simulink model "vocoder_model"  (R2017b)
settings: Solver=VariableStepAuto  StartTime=0.0  StopTime=20  RelTol=1e-3
undefined symbols (not defined in the file or in its folder): NB
libraries: xbsIndex_r4 x1026, dspsrcs4 x1
(part 2 of 8)

== system vocoder_model/Channel_25 ==
  Input : Inport
  Abs Scope : Scope
  Absolute : xbsIndex_r4/Absolute  precision=User Defined  arith_type="Signed  (2's comp)"  n_bits=16  bin_pt=15  quantization=Truncate  overflow=Wrap  en=off  latency=0  dbl_ovrd=off  block_type=abs
  Convert : xbsIndex_r4/Convert  gui_display_data_type=Fixed-point  arith_type="Signed  (2's comp)"  n_bits=16  bin_pt=15  float_type=Single  exp_bits=8  fraction_bits=24  quantization=Truncate  overflow=Wrap  en=off  latency=0  pipeline=off  dbl_ovrd=off  block_type=convert
  Final Channel Scope : Scope
  Gateway In : xbsIndex_r4/Gateway In  gui_display_data_type=Fixed-point  arith_type="Signed  (2's comp)"  n_bits=16  bin_pt=15  preci_type=Single  exp_width=8  frac_width=24  rows=1  columns=1  quantization=Truncate  overflow=Wrap  period=1/8000  UseAsADC=off  ADCChannel='1'  interface=None  automatic_assignment=on  address_offset=hex2dec('00')  intf_name=''  intf_description=''  default_value=0  timing_constraint=None  locs_specified=off  LOCs={}  io_standard={}  inherit_from_input=off  hdl_port=on  dbl_ovrd=off  block_type=gatewayin
  Gateway Out{,1..3} (4 alike) : xbsIndex_r4/Gateway Out  inherit_from_input=off  hdl_port=off  rows=1  columns=1  UseAsDAC=off  DACChannel='1'  interface=None  automatic_assignment=on  address_offset=hex2dec('00')  intf_name=''  intf_description=''  timing_constraint=None  locs_specified=off  LOCs={}  io_standard={}  block_type=gatewayout
  IIR Filter : Subsystem
  IIR Filter Scope : Scope
  LPF Scope : Scope
  Low Pass Filter : Subsystem
  Mult : xbsIndex_r4/Mult  precision=User Defined  arith_type="Signed  (2's comp)"  n_bits=16  bin_pt=15  quantization=Truncate  overflow=Wrap  en=off  latency=0  use_behavioral_HDL=off  opt=Speed  use_embedded=on  optimum_pipeline=off  pipeline=on  dbl_ovrd=off  use_rpm=on  placement_style=Triangular  block_type=mult
  Sine Wave : Sin  Frequency=2*pi*fc  SampleTime=1/8000
  Output : Outport
  wires:
  Input/1 -> IIR Filter/1(Input)
  IIR Filter/1(Output) -> Gateway Out1/1, Absolute/1
  Sine Wave/1 -> Gateway In/1
  Convert/1 -> Mult/1
  Gateway In/1 -> Mult/2
  Absolute/1 -> Gateway Out2/1, Low Pass Filter/1(Input1)
  Low Pass Filter/1(Output1) -> Gateway Out3/1, Convert/1
  Gateway Out/1 -> Output/1, Final Channel Scope/1
  Mult/1 -> Gateway Out/1
  Gateway Out1/1 -> IIR Filter Scope/1
  Gateway Out2/1 -> Abs Scope/1
  Gateway Out3/1 -> LPF Scope/1

== system vocoder_model/Channel_26 ==
  Input : Inport
  Abs Scope : Scope
  Absolute : xbsIndex_r4/Absolute  precision=User Defined  arith_type="Signed  (2's comp)"  n_bits=16  bin_pt=15  quantization=Truncate  overflow=Wrap  en=off  latency=0  dbl_ovrd=off  block_type=abs
  Convert : xbsIndex_r4/Convert  gui_display_data_type=Fixed-point  arith_type="Signed  (2's comp)"  n_bits=16  bin_pt=15  float_type=Single  exp_bits=8  fraction_bits=24  quantization=Truncate  overflow=Wrap  en=off  latency=0  pipeline=off  dbl_ovrd=off  block_type=convert
  Final Channel Scope : Scope
  Gateway In : xbsIndex_r4/Gateway In  gui_display_data_type=Fixed-point  arith_type="Signed  (2's comp)"  n_bits=16  bin_pt=15  preci_type=Single  exp_width=8  frac_width=24  rows=1  columns=1  quantization=Truncate  overflow=Wrap  period=1/8000  UseAsADC=off  ADCChannel='1'  interface=None  automatic_assignment=on  address_offset=hex2dec('00')  intf_name=''  intf_description=''  default_value=0  timing_constraint=None  locs_specified=off  LOCs={}  io_standard={}  inherit_from_input=off  hdl_port=on  dbl_ovrd=off  block_type=gatewayin
  Gateway Out{,1..3} (4 alike) : xbsIndex_r4/Gateway Out  inherit_from_input=off  hdl_port=off  rows=1  columns=1  UseAsDAC=off  DACChannel='1'  interface=None  automatic_assignment=on  address_offset=hex2dec('00')  intf_name=''  intf_description=''  timing_constraint=None  locs_specified=off  LOCs={}  io_standard={}  block_type=gatewayout
  IIR Filter : Subsystem
  IIR Filter Scope : Scope
  LPF Scope : Scope
  Low Pass Filter : Subsystem
  Mult : xbsIndex_r4/Mult  precision=User Defined  arith_type="Signed  (2's comp)"  n_bits=16  bin_pt=15  quantization=Truncate  overflow=Wrap  en=off  latency=0  use_behavioral_HDL=off  opt=Speed  use_embedded=on  optimum_pipeline=off  pipeline=on  dbl_ovrd=off  use_rpm=on  placement_style=Triangular  block_type=mult
  Sine Wave : Sin  Frequency=2*pi*fc  SampleTime=1/8000
  Output : Outport
  wires:
  Input/1 -> IIR Filter/1(Input)
  IIR Filter/1(Output) -> Gateway Out1/1, Absolute/1
  Sine Wave/1 -> Gateway In/1
  Convert/1 -> Mult/1
  Gateway In/1 -> Mult/2
  Absolute/1 -> Gateway Out2/1, Low Pass Filter/1(Input1)
  Low Pass Filter/1(Output1) -> Gateway Out3/1, Convert/1
  Gateway Out/1 -> Output/1, Final Channel Scope/1
  Mult/1 -> Gateway Out/1
  Gateway Out1/1 -> IIR Filter Scope/1
  Gateway Out2/1 -> Abs Scope/1
  Gateway Out3/1 -> LPF Scope/1

== system vocoder_model/Channel_27 ==
  Input : Inport
  Abs Scope : Scope
  Absolute : xbsIndex_r4/Absolute  precision=User Defined  arith_type="Signed  (2's comp)"  n_bits=16  bin_pt=15  quantization=Truncate  overflow=Wrap  en=off  latency=0  dbl_ovrd=off  block_type=abs
  Convert : xbsIndex_r4/Convert  gui_display_data_type=Fixed-point  arith_type="Signed  (2's comp)"  n_bits=16  bin_pt=15  float_type=Single  exp_bits=8  fraction_bits=24  quantization=Truncate  overflow=Wrap  en=off  latency=0  pipeline=off  dbl_ovrd=off  block_type=convert
  Final Channel Scope : Scope
  Gateway In : xbsIndex_r4/Gateway In  gui_display_data_type=Fixed-point  arith_type="Signed  (2's comp)"  n_bits=16  bin_pt=15  preci_type=Single  exp_width=8  frac_width=24  rows=1  columns=1  quantization=Truncate  overflow=Wrap  period=1/8000  UseAsADC=off  ADCChannel='1'  interface=None  automatic_assignment=on  address_offset=hex2dec('00')  intf_name=''  intf_description=''  default_value=0  timing_constraint=None  locs_specified=off  LOCs={}  io_standard={}  inherit_from_input=off  hdl_port=on  dbl_ovrd=off  block_type=gatewayin
  Gateway Out{,1..3} (4 alike) : xbsIndex_r4/Gateway Out  inherit_from_input=off  hdl_port=off  rows=1  columns=1  UseAsDAC=off  DACChannel='1'  interface=None  automatic_assignment=on  address_offset=hex2dec('00')  intf_name=''  intf_description=''  timing_constraint=None  locs_specified=off  LOCs={}  io_standard={}  block_type=gatewayout
  IIR Filter : Subsystem
  IIR Filter Scope : Scope
  LPF Scope : Scope
  Low Pass Filter : Subsystem
  Mult : xbsIndex_r4/Mult  precision=User Defined  arith_type="Signed  (2's comp)"  n_bits=16  bin_pt=15  quantization=Truncate  overflow=Wrap  en=off  latency=0  use_behavioral_HDL=off  opt=Speed  use_embedded=on  optimum_pipeline=off  pipeline=on  dbl_ovrd=off  use_rpm=on  placement_style=Triangular  block_type=mult
  Sine Wave : Sin  Frequency=2*pi*fc  SampleTime=1/8000
  Output : Outport
  wires:
  Input/1 -> IIR Filter/1(Input)
  IIR Filter/1(Output) -> Gateway Out1/1, Absolute/1
  Sine Wave/1 -> Gateway In/1
  Convert/1 -> Mult/1
  Gateway In/1 -> Mult/2
  Absolute/1 -> Gateway Out2/1, Low Pass Filter/1(Input1)
  Low Pass Filter/1(Output1) -> Gateway Out3/1, Convert/1
  Gateway Out/1 -> Output/1, Final Channel Scope/1
  Mult/1 -> Gateway Out/1
  Gateway Out1/1 -> IIR Filter Scope/1
  Gateway Out2/1 -> Abs Scope/1
  Gateway Out3/1 -> LPF Scope/1

== system vocoder_model/Channel_28 ==
  Input : Inport
  Abs Scope : Scope
  Absolute : xbsIndex_r4/Absolute  precision=User Defined  arith_type="Signed  (2's comp)"  n_bits=16  bin_pt=15  quantization=Truncate  overflow=Wrap  en=off  latency=0  dbl_ovrd=off  block_type=abs
  Convert : xbsIndex_r4/Convert  gui_display_data_type=Fixed-point  arith_type="Signed  (2's comp)"  n_bits=16  bin_pt=15  float_type=Single  exp_bits=8  fraction_bits=24  quantization=Truncate  overflow=Wrap  en=off  latency=0  pipeline=off  dbl_ovrd=off  block_type=convert
  Final Channel Scope : Scope
  Gateway In : xbsIndex_r4/Gateway In  gui_display_data_type=Fixed-point  arith_type="Signed  (2's comp)"  n_bits=16  bin_pt=15  preci_type=Single  exp_width=8  frac_width=24  rows=1  columns=1  quantization=Truncate  overflow=Wrap  period=1/8000  UseAsADC=off  ADCChannel='1'  interface=None  automatic_assignment=on  address_offset=hex2dec('00')  intf_name=''  intf_description=''  default_value=0  timing_constraint=None  locs_specified=off  LOCs={}  io_standard={}  inherit_from_input=off  hdl_port=on  dbl_ovrd=off  block_type=gatewayin
  Gateway Out{,1..3} (4 alike) : xbsIndex_r4/Gateway Out  inherit_from_input=off  hdl_port=off  rows=1  columns=1  UseAsDAC=off  DACChannel='1'  interface=None  automatic_assignment=on  address_offset=hex2dec('00')  intf_name=''  intf_description=''  timing_constraint=None  locs_specified=off  LOCs={}  io_standard={}  block_type=gatewayout
  IIR Filter : Subsystem
  IIR Filter Scope : Scope
  LPF Scope : Scope
  Low Pass Filter : Subsystem
  Mult : xbsIndex_r4/Mult  precision=User Defined  arith_type="Signed  (2's comp)"  n_bits=16  bin_pt=15  quantization=Truncate  overflow=Wrap  en=off  latency=0  use_behavioral_HDL=off  opt=Speed  use_embedded=on  optimum_pipeline=off  pipeline=on  dbl_ovrd=off  use_rpm=on  placement_style=Triangular  block_type=mult
  Sine Wave : Sin  Frequency=2*pi*fc  SampleTime=1/8000
  Output : Outport
  wires:
  Input/1 -> IIR Filter/1(Input)
  IIR Filter/1(Output) -> Gateway Out1/1, Absolute/1
  Sine Wave/1 -> Gateway In/1
  Convert/1 -> Mult/1
  Gateway In/1 -> Mult/2
  Absolute/1 -> Gateway Out2/1, Low Pass Filter/1(Input1)
  Low Pass Filter/1(Output1) -> Gateway Out3/1, Convert/1
  Gateway Out/1 -> Output/1, Final Channel Scope/1
  Mult/1 -> Gateway Out/1
  Gateway Out1/1 -> IIR Filter Scope/1
  Gateway Out2/1 -> Abs Scope/1
  Gateway Out3/1 -> LPF Scope/1

== system vocoder_model/Channel_29 ==
  Input : Inport
  Abs Scope : Scope
  Absolute : xbsIndex_r4/Absolute  precision=User Defined  arith_type="Signed  (2's comp)"  n_bits=16  bin_pt=15  quantization=Truncate  overflow=Wrap  en=off  latency=0  dbl_ovrd=off  block_type=abs
  Convert : xbsIndex_r4/Convert  gui_display_data_type=Fixed-point  arith_type="Signed  (2's comp)"  n_bits=16  bin_pt=15  float_type=Single  exp_bits=8  fraction_bits=24  quantization=Truncate  overflow=Wrap  en=off  latency=0  pipeline=off  dbl_ovrd=off  block_type=convert
  Final Channel Scope : Scope
  Gateway In : xbsIndex_r4/Gateway In  gui_display_data_type=Fixed-point  arith_type="Signed  (2's comp)"  n_bits=16  bin_pt=15  preci_type=Single  exp_width=8  frac_width=24  rows=1  columns=1  quantization=Truncate  overflow=Wrap  period=1/8000  UseAsADC=off  ADCChannel='1'  interface=None  automatic_assignment=on  address_offset=hex2dec('00')  intf_name=''  intf_description=''  default_value=0  timing_constraint=None  locs_specified=off  LOCs={}  io_standard={}  inherit_from_input=off  hdl_port=on  dbl_ovrd=off  block_type=gatewayin
  Gateway Out{,1..3} (4 alike) : xbsIndex_r4/Gateway Out  inherit_from_input=off  hdl_port=off  rows=1  columns=1  UseAsDAC=off  DACChannel='1'  interface=None  automatic_assignment=on  address_offset=hex2dec('00')  intf_name=''  intf_description=''  timing_constraint=None  locs_specified=off  LOCs={}  io_standard={}  block_type=gatewayout
  IIR Filter : Subsystem
  IIR Filter Scope : Scope
  LPF Scope : Scope
  Low Pass Filter : Subsystem
  Mult : xbsIndex_r4/Mult  precision=User Defined  arith_type="Signed  (2's comp)"  n_bits=16  bin_pt=15  quantization=Truncate  overflow=Wrap  en=off  latency=0  use_behavioral_HDL=off  opt=Speed  use_embedded=on  optimum_pipeline=off  pipeline=on  dbl_ovrd=off  use_rpm=on  placement_style=Triangular  block_type=mult
  Sine Wave : Sin  Frequency=2*pi*fc  SampleTime=1/8000
  Output : Outport
  wires:
  Input/1 -> IIR Filter/1(Input)
  IIR Filter/1(Output) -> Gateway Out1/1, Absolute/1
  Sine Wave/1 -> Gateway In/1
  Convert/1 -> Mult/1
  Gateway In/1 -> Mult/2
  Absolute/1 -> Gateway Out2/1, Low Pass Filter/1(Input1)
  Low Pass Filter/1(Output1) -> Gateway Out3/1, Convert/1
  Gateway Out/1 -> Output/1, Final Channel Scope/1
  Mult/1 -> Gateway Out/1
  Gateway Out1/1 -> IIR Filter Scope/1
  Gateway Out2/1 -> Abs Scope/1
  Gateway Out3/1 -> LPF Scope/1

== system vocoder_model/Channel_3 ==
  Input : Inport
  Abs Scope : Scope
  Absolute : xbsIndex_r4/Absolute  precision=User Defined  arith_type="Signed  (2's comp)"  n_bits=16  bin_pt=15  quantization=Truncate  overflow=Wrap  en=off  latency=0  dbl_ovrd=off  block_type=abs
  Convert : xbsIndex_r4/Convert  gui_display_data_type=Fixed-point  arith_type="Signed  (2's comp)"  n_bits=16  bin_pt=15  float_type=Single  exp_bits=8  fraction_bits=24  quantization=Truncate  overflow=Wrap  en=off  latency=0  pipeline=off  dbl_ovrd=off  block_type=convert
  Final Channel Scope : Scope
  Gateway In : xbsIndex_r4/Gateway In  gui_display_data_type=Fixed-point  arith_type="Signed  (2's comp)"  n_bits=16  bin_pt=15  preci_type=Single  exp_width=8  frac_width=24  rows=1  columns=1  quantization=Truncate  overflow=Wrap  period=1/8000  UseAsADC=off  ADCChannel='1'  interface=None  automatic_assignment=on  address_offset=hex2dec('00')  intf_name=''  intf_description=''  default_value=0  timing_constraint=None  locs_specified=off  LOCs={}  io_standard={}  inherit_from_input=off  hdl_port=on  dbl_ovrd=off  block_type=gatewayin
  Gateway Out{,1..3} (4 alike) : xbsIndex_r4/Gateway Out  inherit_from_input=off  hdl_port=off  rows=1  columns=1  UseAsDAC=off  DACChannel='1'  interface=None  automatic_assignment=on  address_offset=hex2dec('00')  intf_name=''  intf_description=''  timing_constraint=None  locs_specified=off  LOCs={}  io_standard={}  block_type=gatewayout
  IIR Filter : Subsystem
  IIR Filter Scope : Scope
  LPF Scope : Scope
  Low Pass Filter : Subsystem
  Mult : xbsIndex_r4/Mult  precision=User Defined  arith_type="Signed  (2's comp)"  n_bits=16  bin_pt=15  quantization=Truncate  overflow=Wrap  en=off  latency=0  use_behavioral_HDL=off  opt=Speed  use_embedded=on  optimum_pipeline=off  pipeline=on  dbl_ovrd=off  use_rpm=on  placement_style=Triangular  block_type=mult
  Sine Wave : Sin  Frequency=2*pi*fc  SampleTime=1/8000
  Output : Outport
  wires:
  Input/1 -> IIR Filter/1(Input)
  IIR Filter/1(Output) -> Gateway Out1/1, Absolute/1
  Sine Wave/1 -> Gateway In/1
  Convert/1 -> Mult/1
  Gateway In/1 -> Mult/2
  Absolute/1 -> Gateway Out2/1, Low Pass Filter/1(Input1)
  Low Pass Filter/1(Output1) -> Gateway Out3/1, Convert/1
  Gateway Out/1 -> Output/1, Final Channel Scope/1
  Mult/1 -> Gateway Out/1
  Gateway Out1/1 -> IIR Filter Scope/1
  Gateway Out2/1 -> Abs Scope/1
  Gateway Out3/1 -> LPF Scope/1

== system vocoder_model/Channel_30 ==
  Input : Inport
  Abs Scope : Scope
  Absolute : xbsIndex_r4/Absolute  precision=User Defined  arith_type="Signed  (2's comp)"  n_bits=16  bin_pt=15  quantization=Truncate  overflow=Wrap  en=off  latency=0  dbl_ovrd=off  block_type=abs
  Convert : xbsIndex_r4/Convert  gui_display_data_type=Fixed-point  arith_type="Signed  (2's comp)"  n_bits=16  bin_pt=15  float_type=Single  exp_bits=8  fraction_bits=24  quantization=Truncate  overflow=Wrap  en=off  latency=0  pipeline=off  dbl_ovrd=off  block_type=convert
  Final Channel Scope : Scope
  Gateway In : xbsIndex_r4/Gateway In  gui_display_data_type=Fixed-point  arith_type="Signed  (2's comp)"  n_bits=16  bin_pt=15  preci_type=Single  exp_width=8  frac_width=24  rows=1  columns=1  quantization=Truncate  overflow=Wrap  period=1/8000  UseAsADC=off  ADCChannel='1'  interface=None  automatic_assignment=on  address_offset=hex2dec('00')  intf_name=''  intf_description=''  default_value=0  timing_constraint=None  locs_specified=off  LOCs={}  io_standard={}  inherit_from_input=off  hdl_port=on  dbl_ovrd=off  block_type=gatewayin
  Gateway Out{,1..3} (4 alike) : xbsIndex_r4/Gateway Out  inherit_from_input=off  hdl_port=off  rows=1  columns=1  UseAsDAC=off  DACChannel='1'  interface=None  automatic_assignment=on  address_offset=hex2dec('00')  intf_name=''  intf_description=''  timing_constraint=None  locs_specified=off  LOCs={}  io_standard={}  block_type=gatewayout
  IIR Filter : Subsystem
  IIR Filter Scope : Scope
  LPF Scope : Scope
  Low Pass Filter : Subsystem
  Mult : xbsIndex_r4/Mult  precision=User Defined  arith_type="Signed  (2's comp)"  n_bits=16  bin_pt=15  quantization=Truncate  overflow=Wrap  en=off  latency=0  use_behavioral_HDL=off  opt=Speed  use_embedded=on  optimum_pipeline=off  pipeline=on  dbl_ovrd=off  use_rpm=on  placement_style=Triangular  block_type=mult
  Sine Wave : Sin  Frequency=2*pi*fc  SampleTime=1/8000
  Output : Outport
  wires:
  Input/1 -> IIR Filter/1(Input)
  IIR Filter/1(Output) -> Gateway Out1/1, Absolute/1
  Sine Wave/1 -> Gateway In/1
  Convert/1 -> Mult/1
  Gateway In/1 -> Mult/2
  Absolute/1 -> Gateway Out2/1, Low Pass Filter/1(Input1)
  Low Pass Filter/1(Output1) -> Gateway Out3/1, Convert/1
  Gateway Out/1 -> Output/1, Final Channel Scope/1
  Mult/1 -> Gateway Out/1
  Gateway Out1/1 -> IIR Filter Scope/1
  Gateway Out2/1 -> Abs Scope/1
  Gateway Out3/1 -> LPF Scope/1

== system vocoder_model/Channel_31 ==
  Input : Inport
  Abs Scope : Scope
  Absolute : xbsIndex_r4/Absolute  precision=User Defined  arith_type="Signed  (2's comp)"  n_bits=16  bin_pt=15  quantization=Truncate  overflow=Wrap  en=off  latency=0  dbl_ovrd=off  block_type=abs
  Convert : xbsIndex_r4/Convert  gui_display_data_type=Fixed-point  arith_type="Signed  (2's comp)"  n_bits=16  bin_pt=15  float_type=Single  exp_bits=8  fraction_bits=24  quantization=Truncate  overflow=Wrap  en=off  latency=0  pipeline=off  dbl_ovrd=off  block_type=convert
  Final Channel Scope : Scope
  Gateway In : xbsIndex_r4/Gateway In  gui_display_data_type=Fixed-point  arith_type="Signed  (2's comp)"  n_bits=16  bin_pt=15  preci_type=Single  exp_width=8  frac_width=24  rows=1  columns=1  quantization=Truncate  overflow=Wrap  period=1/8000  UseAsADC=off  ADCChannel='1'  interface=None  automatic_assignment=on  address_offset=hex2dec('00')  intf_name=''  intf_description=''  default_value=0  timing_constraint=None  locs_specified=off  LOCs={}  io_standard={}  inherit_from_input=off  hdl_port=on  dbl_ovrd=off  block_type=gatewayin
  Gateway Out{,1..3} (4 alike) : xbsIndex_r4/Gateway Out  inherit_from_input=off  hdl_port=off  rows=1  columns=1  UseAsDAC=off  DACChannel='1'  interface=None  automatic_assignment=on  address_offset=hex2dec('00')  intf_name=''  intf_description=''  timing_constraint=None  locs_specified=off  LOCs={}  io_standard={}  block_type=gatewayout
  IIR Filter : Subsystem
  IIR Filter Scope : Scope
  LPF Scope : Scope
  Low Pass Filter : Subsystem
  Mult : xbsIndex_r4/Mult  precision=User Defined  arith_type="Signed  (2's comp)"  n_bits=16  bin_pt=15  quantization=Truncate  overflow=Wrap  en=off  latency=0  use_behavioral_HDL=off  opt=Speed  use_embedded=on  optimum_pipeline=off  pipeline=on  dbl_ovrd=off  use_rpm=on  placement_style=Triangular  block_type=mult
  Sine Wave : Sin  Frequency=2*pi*fc  SampleTime=1/8000
  Output : Outport
  wires:
  Input/1 -> IIR Filter/1(Input)
  IIR Filter/1(Output) -> Gateway Out1/1, Absolute/1
  Sine Wave/1 -> Gateway In/1
  Convert/1 -> Mult/1
  Gateway In/1 -> Mult/2
  Absolute/1 -> Gateway Out2/1, Low Pass Filter/1(Input1)
  Low Pass Filter/1(Output1) -> Gateway Out3/1, Convert/1
  Gateway Out/1 -> Output/1, Final Channel Scope/1
  Mult/1 -> Gateway Out/1
  Gateway Out1/1 -> IIR Filter Scope/1
  Gateway Out2/1 -> Abs Scope/1
  Gateway Out3/1 -> LPF Scope/1

== system vocoder_model/Channel_32 ==
  Input : Inport
  Abs Scope : Scope
  Absolute : xbsIndex_r4/Absolute  precision=User Defined  arith_type="Signed  (2's comp)"  n_bits=16  bin_pt=15  quantization=Truncate  overflow=Wrap  en=off  latency=0  dbl_ovrd=off  block_type=abs
  Convert : xbsIndex_r4/Convert  gui_display_data_type=Fixed-point  arith_type="Signed  (2's comp)"  n_bits=16  bin_pt=15  float_type=Single  exp_bits=8  fraction_bits=24  quantization=Truncate  overflow=Wrap  en=off  latency=0  pipeline=off  dbl_ovrd=off  block_type=convert
  Final Channel Scope : Scope
  Gateway In : xbsIndex_r4/Gateway In  gui_display_data_type=Fixed-point  arith_type="Signed  (2's comp)"  n_bits=16  bin_pt=15  preci_type=Single  exp_width=8  frac_width=24  rows=1  columns=1  quantization=Truncate  overflow=Wrap  period=1/8000  UseAsADC=off  ADCChannel='1'  interface=None  automatic_assignment=on  address_offset=hex2dec('00')  intf_name=''  intf_description=''  default_value=0  timing_constraint=None  locs_specified=off  LOCs={}  io_standard={}  inherit_from_input=off  hdl_port=on  dbl_ovrd=off  block_type=gatewayin
  Gateway Out{,1..3} (4 alike) : xbsIndex_r4/Gateway Out  inherit_from_input=off  hdl_port=off  rows=1  columns=1  UseAsDAC=off  DACChannel='1'  interface=None  automatic_assignment=on  address_offset=hex2dec('00')  intf_name=''  intf_description=''  timing_constraint=None  locs_specified=off  LOCs={}  io_standard={}  block_type=gatewayout
  IIR Filter : Subsystem
  IIR Filter Scope : Scope
  LPF Scope : Scope
  Low Pass Filter : Subsystem
  Mult : xbsIndex_r4/Mult  precision=User Defined  arith_type="Signed  (2's comp)"  n_bits=16  bin_pt=15  quantization=Truncate  overflow=Wrap  en=off  latency=0  use_behavioral_HDL=off  opt=Speed  use_embedded=on  optimum_pipeline=off  pipeline=on  dbl_ovrd=off  use_rpm=on  placement_style=Triangular  block_type=mult
  Sine Wave : Sin  Frequency=2*pi*fc  SampleTime=1/8000
  Output : Outport
  wires:
  Input/1 -> IIR Filter/1(Input)
  IIR Filter/1(Output) -> Gateway Out1/1, Absolute/1
  Sine Wave/1 -> Gateway In/1
  Convert/1 -> Mult/1
  Gateway In/1 -> Mult/2
  Absolute/1 -> Gateway Out2/1, Low Pass Filter/1(Input1)
  Low Pass Filter/1(Output1) -> Gateway Out3/1, Convert/1
  Gateway Out/1 -> Output/1, Final Channel Scope/1
  Mult/1 -> Gateway Out/1
  Gateway Out1/1 -> IIR Filter Scope/1
  Gateway Out2/1 -> Abs Scope/1
  Gateway Out3/1 -> LPF Scope/1

== system vocoder_model/Channel_4 ==
  Input : Inport
  Abs Scope : Scope
  Absolute : xbsIndex_r4/Absolute  precision=User Defined  arith_type="Signed  (2's comp)"  n_bits=16  bin_pt=15  quantization=Truncate  overflow=Wrap  en=off  latency=0  dbl_ovrd=off  block_type=abs
  Convert : xbsIndex_r4/Convert  gui_display_data_type=Fixed-point  arith_type="Signed  (2's comp)"  n_bits=16  bin_pt=15  float_type=Single  exp_bits=8  fraction_bits=24  quantization=Truncate  overflow=Wrap  en=off  latency=0  pipeline=off  dbl_ovrd=off  block_type=convert
  Final Channel Scope : Scope
  Gateway In : xbsIndex_r4/Gateway In  gui_display_data_type=Fixed-point  arith_type="Signed  (2's comp)"  n_bits=16  bin_pt=15  preci_type=Single  exp_width=8  frac_width=24  rows=1  columns=1  quantization=Truncate  overflow=Wrap  period=1/8000  UseAsADC=off  ADCChannel='1'  interface=None  automatic_assignment=on  address_offset=hex2dec('00')  intf_name=''  intf_description=''  default_value=0  timing_constraint=None  locs_specified=off  LOCs={}  io_standard={}  inherit_from_input=off  hdl_port=on  dbl_ovrd=off  block_type=gatewayin
  Gateway Out{,1..3} (4 alike) : xbsIndex_r4/Gateway Out  inherit_from_input=off  hdl_port=off  rows=1  columns=1  UseAsDAC=off  DACChannel='1'  interface=None  automatic_assignment=on  address_offset=hex2dec('00')  intf_name=''  intf_description=''  timing_constraint=None  locs_specified=off  LOCs={}  io_standard={}  block_type=gatewayout
  IIR Filter : Subsystem
  IIR Filter Scope : Scope
  LPF Scope : Scope
  Low Pass Filter : Subsystem
  Mult : xbsIndex_r4/Mult  precision=User Defined  arith_type="Signed  (2's comp)"  n_bits=16  bin_pt=15  quantization=Truncate  overflow=Wrap  en=off  latency=0  use_behavioral_HDL=off  opt=Speed  use_embedded=on  optimum_pipeline=off  pipeline=on  dbl_ovrd=off  use_rpm=on  placement_style=Triangular  block_type=mult
  Sine Wave : Sin  Frequency=2*pi*fc  SampleTime=1/8000
  Output : Outport
  wires:
  Input/1 -> IIR Filter/1(Input)
  IIR Filter/1(Output) -> Gateway Out1/1, Absolute/1
  Sine Wave/1 -> Gateway In/1
  Convert/1 -> Mult/1
  Gateway In/1 -> Mult/2
  Absolute/1 -> Gateway Out2/1, Low Pass Filter/1(Input1)
  Low Pass Filter/1(Output1) -> Gateway Out3/1, Convert/1
  Gateway Out/1 -> Output/1, Final Channel Scope/1
  Mult/1 -> Gateway Out/1
  Gateway Out1/1 -> IIR Filter Scope/1
  Gateway Out2/1 -> Abs Scope/1
  Gateway Out3/1 -> LPF Scope/1

== system vocoder_model/Channel_5 ==
  Input : Inport
  Abs Scope : Scope
  Absolute : xbsIndex_r4/Absolute  precision=User Defined  arith_type="Signed  (2's comp)"  n_bits=16  bin_pt=15  quantization=Truncate  overflow=Wrap  en=off  latency=0  dbl_ovrd=off  block_type=abs
  Convert : xbsIndex_r4/Convert  gui_display_data_type=Fixed-point  arith_type="Signed  (2's comp)"  n_bits=16  bin_pt=15  float_type=Single  exp_bits=8  fraction_bits=24  quantization=Truncate  overflow=Wrap  en=off  latency=0  pipeline=off  dbl_ovrd=off  block_type=convert
  Final Channel Scope : Scope
  Gateway In : xbsIndex_r4/Gateway In  gui_display_data_type=Fixed-point  arith_type="Signed  (2's comp)"  n_bits=16  bin_pt=15  preci_type=Single  exp_width=8  frac_width=24  rows=1  columns=1  quantization=Truncate  overflow=Wrap  period=1/8000  UseAsADC=off  ADCChannel='1'  interface=None  automatic_assignment=on  address_offset=hex2dec('00')  intf_name=''  intf_description=''  default_value=0  timing_constraint=None  locs_specified=off  LOCs={}  io_standard={}  inherit_from_input=off  hdl_port=on  dbl_ovrd=off  block_type=gatewayin
  Gateway Out{,1..3} (4 alike) : xbsIndex_r4/Gateway Out  inherit_from_input=off  hdl_port=off  rows=1  columns=1  UseAsDAC=off  DACChannel='1'  interface=None  automatic_assignment=on  address_offset=hex2dec('00')  intf_name=''  intf_description=''  timing_constraint=None  locs_specified=off  LOCs={}  io_standard={}  block_type=gatewayout
  IIR Filter : Subsystem
  IIR Filter Scope : Scope
  LPF Scope : Scope
  Low Pass Filter : Subsystem
  Mult : xbsIndex_r4/Mult  precision=User Defined  arith_type="Signed  (2's comp)"  n_bits=16  bin_pt=15  quantization=Truncate  overflow=Wrap  en=off  latency=0  use_behavioral_HDL=off  opt=Speed  use_embedded=on  optimum_pipeline=off  pipeline=on  dbl_ovrd=off  use_rpm=on  placement_style=Triangular  block_type=mult
  Sine Wave : Sin  Frequency=2*pi*fc  SampleTime=1/8000
  Output : Outport
  wires:
  Input/1 -> IIR Filter/1(Input)
  IIR Filter/1(Output) -> Gateway Out1/1, Absolute/1
  Sine Wave/1 -> Gateway In/1
  Convert/1 -> Mult/1
  Gateway In/1 -> Mult/2
  Absolute/1 -> Gateway Out2/1, Low Pass Filter/1(Input1)
  Low Pass Filter/1(Output1) -> Gateway Out3/1, Convert/1
  Gateway Out/1 -> Output/1, Final Channel Scope/1
  Mult/1 -> Gateway Out/1
  Gateway Out1/1 -> IIR Filter Scope/1
  Gateway Out2/1 -> Abs Scope/1
  Gateway Out3/1 -> LPF Scope/1

== system vocoder_model/Channel_6 ==
  Input : Inport
  Abs Scope : Scope
  Absolute : xbsIndex_r4/Absolute  precision=User Defined  arith_type="Signed  (2's comp)"  n_bits=16  bin_pt=15  quantization=Truncate  overflow=Wrap  en=off  latency=0  dbl_ovrd=off  block_type=abs
  Convert : xbsIndex_r4/Convert  gui_display_data_type=Fixed-point  arith_type="Signed  (2's comp)"  n_bits=16  bin_pt=15  float_type=Single  exp_bits=8  fraction_bits=24  quantization=Truncate  overflow=Wrap  en=off  latency=0  pipeline=off  dbl_ovrd=off  block_type=convert
  Final Channel Scope : Scope
  Gateway In : xbsIndex_r4/Gateway In  gui_display_data_type=Fixed-point  arith_type="Signed  (2's comp)"  n_bits=16  bin_pt=15  preci_type=Single  exp_width=8  frac_width=24  rows=1  columns=1  quantization=Truncate  overflow=Wrap  period=1/8000  UseAsADC=off  ADCChannel='1'  interface=None  automatic_assignment=on  address_offset=hex2dec('00')  intf_name=''  intf_description=''  default_value=0  timing_constraint=None  locs_specified=off  LOCs={}  io_standard={}  inherit_from_input=off  hdl_port=on  dbl_ovrd=off  block_type=gatewayin
  Gateway Out{,1..3} (4 alike) : xbsIndex_r4/Gateway Out  inherit_from_input=off  hdl_port=off  rows=1  columns=1  UseAsDAC=off  DACChannel='1'  interface=None  automatic_assignment=on  address_offset=hex2dec('00')  intf_name=''  intf_description=''  timing_constraint=None  locs_specified=off  LOCs={}  io_standard={}  block_type=gatewayout
  IIR Filter : Subsystem
  IIR Filter Scope : Scope
  LPF Scope : Scope
  Low Pass Filter : Subsystem
  Mult : xbsIndex_r4/Mult  precision=User Defined  arith_type="Signed  (2's comp)"  n_bits=16  bin_pt=15  quantization=Truncate  overflow=Wrap  en=off  latency=0  use_behavioral_HDL=off  opt=Speed  use_embedded=on  optimum_pipeline=off  pipeline=on  dbl_ovrd=off  use_rpm=on  placement_style=Triangular  block_type=mult
  Sine Wave : Sin  Frequency=2*pi*fc  SampleTime=1/8000
  Output : Outport
  wires:
  Input/1 -> IIR Filter/1(Input)
  IIR Filter/1(Output) -> Gateway Out1/1, Absolute/1
  Sine Wave/1 -> Gateway In/1
  Convert/1 -> Mult/1
  Gateway In/1 -> Mult/2
  Absolute/1 -> Gateway Out2/1, Low Pass Filter/1(Input1)
  Low Pass Filter/1(Output1) -> Gateway Out3/1, Convert/1
  Gateway Out/1 -> Output/1, Final Channel Scope/1
  Mult/1 -> Gateway Out/1
  Gateway Out1/1 -> IIR Filter Scope/1
  Gateway Out2/1 -> Abs Scope/1
  Gateway Out3/1 -> LPF Scope/1

== system vocoder_model/Channel_7 ==
  Input : Inport
  Abs Scope : Scope
  Absolute : xbsIndex_r4/Absolute  precision=User Defined  arith_type="Signed  (2's comp)"  n_bits=16  bin_pt=15  quantization=Truncate  overflow=Wrap  en=off  latency=0  dbl_ovrd=off  block_type=abs
  Convert : xbsIndex_r4/Convert  gui_display_data_type=Fixed-point  arith_type="Signed  (2's comp)"  n_bits=16  bin_pt=15  float_type=Single  exp_bits=8  fraction_bits=24  quantization=Truncate  overflow=Wrap  en=off  latency=0  pipeline=off  dbl_ovrd=off  block_type=convert
  Final Channel Scope : Scope
  Gateway In : xbsIndex_r4/Gateway In  gui_display_data_type=Fixed-point  arith_type="Signed  (2's comp)"  n_bits=16  bin_pt=15  preci_type=Single  exp_width=8  frac_width=24  rows=1  columns=1  quantization=Truncate  overflow=Wrap  period=1/8000  UseAsADC=off  ADCChannel='1'  interface=None  automatic_assignment=on  address_offset=hex2dec('00')  intf_name=''  intf_description=''  default_value=0  timing_constraint=None  locs_specified=off  LOCs={}  io_standard={}  inherit_from_input=off  hdl_port=on  dbl_ovrd=off  block_type=gatewayin
  Gateway Out{,1..3} (4 alike) : xbsIndex_r4/Gateway Out  inherit_from_input=off  hdl_port=off  rows=1  columns=1  UseAsDAC=off  DACChannel='1'  interface=None  automatic_assignment=on  address_offset=hex2dec('00')  intf_name=''  intf_description=''  timing_constraint=None  locs_specified=off  LOCs={}  io_standard={}  block_type=gatewayout
  IIR Filter : Subsystem
  IIR Filter Scope : Scope
  LPF Scope : Scope
  Low Pass Filter : Subsystem
  Mult : xbsIndex_r4/Mult  precision=User Defined  arith_type="Signed  (2's comp)"  n_bits=16  bin_pt=15  quantization=Truncate  overflow=Wrap  en=off  latency=0  use_behavioral_HDL=off  opt=Speed  use_embedded=on  optimum_pipeline=off  pipeline=on  dbl_ovrd=off  use_rpm=on  placement_style=Triangular  block_type=mult
  Sine Wave : Sin  Frequency=2*pi*fc  SampleTime=1/8000
  Output : Outport
  wires:
  Input/1 -> IIR Filter/1(Input)
  IIR Filter/1(Output) -> Gateway Out1/1, Absolute/1
  Sine Wave/1 -> Gateway In/1
  Convert/1 -> Mult/1
  Gateway In/1 -> Mult/2
  Absolute/1 -> Gateway Out2/1, Low Pass Filter/1(Input1)
  Low Pass Filter/1(Output1) -> Gateway Out3/1, Convert/1
  Gateway Out/1 -> Output/1, Final Channel Scope/1
  Mult/1 -> Gateway Out/1
  Gateway Out1/1 -> IIR Filter Scope/1
  Gateway Out2/1 -> Abs Scope/1
  Gateway Out3/1 -> LPF Scope/1

== system vocoder_model/Channel_8 ==
  Input : Inport
  Abs Scope : Scope
  Absolute : xbsIndex_r4/Absolute  precision=User Defined  arith_type="Signed  (2's comp)"  n_bits=16  bin_pt=15  quantization=Truncate  overflow=Wrap  en=off  latency=0  dbl_ovrd=off  block_type=abs
  Convert : xbsIndex_r4/Convert  gui_display_data_type=Fixed-point  arith_type="Signed  (2's comp)"  n_bits=16  bin_pt=15  float_type=Single  exp_bits=8  fraction_bits=24  quantization=Truncate  overflow=Wrap  en=off  latency=0  pipeline=off  dbl_ovrd=off  block_type=convert
  Final Channel Scope : Scope
  Gateway In : xbsIndex_r4/Gateway In  gui_display_data_type=Fixed-point  arith_type="Signed  (2's comp)"  n_bits=16  bin_pt=15  preci_type=Single  exp_width=8  frac_width=24  rows=1  columns=1  quantization=Truncate  overflow=Wrap  period=1/8000  UseAsADC=off  ADCChannel='1'  interface=None  automatic_assignment=on  address_offset=hex2dec('00')  intf_name=''  intf_description=''  default_value=0  timing_constraint=None  locs_specified=off  LOCs={}  io_standard={}  inherit_from_input=off  hdl_port=on  dbl_ovrd=off  block_type=gatewayin
  Gateway Out{,1..3} (4 alike) : xbsIndex_r4/Gateway Out  inherit_from_input=off  hdl_port=off  rows=1  columns=1  UseAsDAC=off  DACChannel='1'  interface=None  automatic_assignment=on  address_offset=hex2dec('00')  intf_name=''  intf_description=''  timing_constraint=None  locs_specified=off  LOCs={}  io_standard={}  block_type=gatewayout
  IIR Filter : Subsystem
  IIR Filter Scope : Scope
  LPF Scope : Scope
  Low Pass Filter : Subsystem
  Mult : xbsIndex_r4/Mult  precision=User Defined  arith_type="Signed  (2's comp)"  n_bits=16  bin_pt=15  quantization=Truncate  overflow=Wrap  en=off  latency=0  use_behavioral_HDL=off  opt=Speed  use_embedded=on  optimum_pipeline=off  pipeline=on  dbl_ovrd=off  use_rpm=on  placement_style=Triangular  block_type=mult
  Sine Wave : Sin  Frequency=2*pi*fc  SampleTime=1/8000
  Output : Outport
  wires:
  Input/1 -> IIR Filter/1(Input)
  IIR Filter/1(Output) -> Gateway Out1/1, Absolute/1
  Sine Wave/1 -> Gateway In/1
  Convert/1 -> Mult/1
  Gateway In/1 -> Mult/2
  Absolute/1 -> Gateway Out2/1, Low Pass Filter/1(Input1)
  Low Pass Filter/1(Output1) -> Gateway Out3/1, Convert/1
  Gateway Out/1 -> Output/1, Final Channel Scope/1
  Mult/1 -> Gateway Out/1
  Gateway Out1/1 -> IIR Filter Scope/1
  Gateway Out2/1 -> Abs Scope/1
  Gateway Out3/1 -> LPF Scope/1

== system vocoder_model/Channel_9 ==
  Input : Inport
  Abs Scope : Scope
  Absolute : xbsIndex_r4/Absolute  precision=User Defined  arith_type="Signed  (2's comp)"  n_bits=16  bin_pt=15  quantization=Truncate  overflow=Wrap  en=off  latency=0  dbl_ovrd=off  block_type=abs
  Convert : xbsIndex_r4/Convert  gui_display_data_type=Fixed-point  arith_type="Signed  (2's comp)"  n_bits=16  bin_pt=15  float_type=Single  exp_bits=8  fraction_bits=24  quantization=Truncate  overflow=Wrap  en=off  latency=0  pipeline=off  dbl_ovrd=off  block_type=convert
  Final Channel Scope : Scope
  Gateway In : xbsIndex_r4/Gateway In  gui_display_data_type=Fixed-point  arith_type="Signed  (2's comp)"  n_bits=16  bin_pt=15  preci_type=Single  exp_width=8  frac_width=24  rows=1  columns=1  quantization=Truncate  overflow=Wrap  period=1/8000  UseAsADC=off  ADCChannel='1'  interface=None  automatic_assignment=on  address_offset=hex2dec('00')  intf_name=''  intf_description=''  default_value=0  timing_constraint=None  locs_specified=off  LOCs={}  io_standard={}  inherit_from_input=off  hdl_port=on  dbl_ovrd=off  block_type=gatewayin
  Gateway Out{,1..3} (4 alike) : xbsIndex_r4/Gateway Out  inherit_from_input=off  hdl_port=off  rows=1  columns=1  UseAsDAC=off  DACChannel='1'  interface=None  automatic_assignment=on  address_offset=hex2dec('00')  intf_name=''  intf_description=''  timing_constraint=None  locs_specified=off  LOCs={}  io_standard={}  block_type=gatewayout
  IIR Filter : Subsystem
  IIR Filter Scope : Scope
  LPF Scope : Scope
  Low Pass Filter : Subsystem
  Mult : xbsIndex_r4/Mult  precision=User Defined  arith_type="Signed  (2's comp)"  n_bits=16  bin_pt=15  quantization=Truncate  overflow=Wrap  en=off  latency=0  use_behavioral_HDL=off  opt=Speed  use_embedded=on  optimum_pipeline=off  pipeline=on  dbl_ovrd=off  use_rpm=on  placement_style=Triangular  block_type=mult
  Sine Wave : Sin  Frequency=2*pi*fc  SampleTime=1/8000
  Output : Outport
  wires:
  Input/1 -> IIR Filter/1(Input)
  IIR Filter/1(Output) -> Gateway Out1/1, Absolute/1
  Sine Wave/1 -> Gateway In/1
  Convert/1 -> Mult/1
  Gateway In/1 -> Mult/2
  Absolute/1 -> Gateway Out2/1, Low Pass Filter/1(Input1)
  Low Pass Filter/1(Output1) -> Gateway Out3/1, Convert/1
  Gateway Out/1 -> Output/1, Final Channel Scope/1
  Mult/1 -> Gateway Out/1
  Gateway Out1/1 -> IIR Filter Scope/1
  Gateway Out2/1 -> Abs Scope/1
  Gateway Out3/1 -> LPF Scope/1

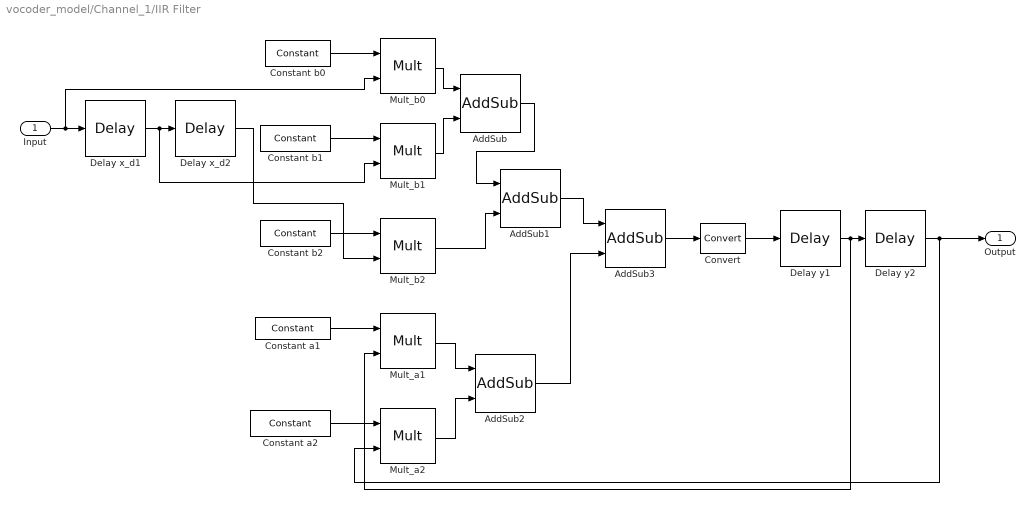
== system vocoder_model/Channel_1/IIR Filter ==
  Input : Inport
  AddSub : xbsIndex_r4/AddSub  mode=Addition  use_carryin=off  use_carryout=off  en=off  latency=0  precision=Full  arith_type=Unsigned  n_bits=16  bin_pt=14  quantization=Truncate  overflow=Wrap  use_behavioral_HDL=off  hw_selection=Fabric  pipelined=off  dbl_ovrd=off  block_type=addsub
  AddSub1 : xbsIndex_r4/AddSub  mode=Addition  use_carryin=off  use_carryout=off  en=off  latency=0  precision=Full  arith_type=Unsigned  n_bits=16  bin_pt=14  quantization=Truncate  overflow=Wrap  use_behavioral_HDL=off  hw_selection=Fabric  pipelined=off  dbl_ovrd=off  block_type=addsub
  AddSub2 : xbsIndex_r4/AddSub  mode=Addition  use_carryin=off  use_carryout=off  en=off  latency=0  precision=Full  arith_type=Unsigned  n_bits=16  bin_pt=14  quantization=Truncate  overflow=Wrap  use_behavioral_HDL=off  hw_selection=Fabric  pipelined=off  dbl_ovrd=off  block_type=addsub
  AddSub3 : xbsIndex_r4/AddSub  mode=Subtraction  use_carryin=off  use_carryout=off  en=off  latency=0  precision=Full  arith_type=Unsigned  n_bits=16  bin_pt=14  quantization=Truncate  overflow=Wrap  use_behavioral_HDL=off  hw_selection=Fabric  pipelined=off  dbl_ovrd=off  block_type=addsub
  Constant a1 : xbsIndex_r4/Constant  const=a1  gui_display_data_type=Fixed-point  arith_type=Signed (2's comp)  n_bits=NB  bin_pt=NB-1  preci_type=Single  exp_width=8  frac_width=24  explicit_period=off  period=1  equ=P=C  opselect=C  inp2=PCIN>>17  opr=+  inp1=P  carry=CIN  dbl_ovrd=off  block_type=constant
  Constant a2 : xbsIndex_r4/Constant  const=a2  gui_display_data_type=Fixed-point  arith_type=Signed (2's comp)  n_bits=NB  bin_pt=NB-1  preci_type=Single  exp_width=8  frac_width=24  explicit_period=off  period=1  equ=P=C  opselect=C  inp2=PCIN>>17  opr=+  inp1=P  carry=CIN  dbl_ovrd=off  block_type=constant
  Constant b0 : xbsIndex_r4/Constant  const=b0  gui_display_data_type=Fixed-point  arith_type=Signed (2's comp)  n_bits=NB  bin_pt=NB-1  preci_type=Single  exp_width=8  frac_width=24  explicit_period=off  period=1  equ=P=C  opselect=C  inp2=PCIN>>17  opr=+  inp1=P  carry=CIN  dbl_ovrd=off  block_type=constant
  Constant b1 : xbsIndex_r4/Constant  const=b1  gui_display_data_type=Fixed-point  arith_type=Signed (2's comp)  n_bits=NB  bin_pt=NB-1  preci_type=Single  exp_width=8  frac_width=24  explicit_period=off  period=1  equ=P=C  opselect=C  inp2=PCIN>>17  opr=+  inp1=P  carry=CIN  dbl_ovrd=off  block_type=constant
  Constant b2 : xbsIndex_r4/Constant  const=b2  gui_display_data_type=Fixed-point  arith_type=Signed (2's comp)  n_bits=NB  bin_pt=NB-1  preci_type=Single  exp_width=8  frac_width=24  explicit_period=off  period=1  equ=P=C  opselect=C  inp2=PCIN>>17  opr=+  inp1=P  carry=CIN  dbl_ovrd=off  block_type=constant
  Convert : xbsIndex_r4/Convert  gui_display_data_type=Fixed-point  arith_type="Signed  (2's comp)"  n_bits=16  bin_pt=15  float_type=Single  exp_bits=8  fraction_bits=24  quantization=Truncate  overflow=Wrap  en=off  latency=0  pipeline=off  dbl_ovrd=off  block_type=convert
  Delay x_d1 : xbsIndex_r4/Delay  rst=off  infoeditControl=Selection of Reset will increase slice count due to use of real FFs and instead of SRLs  en=off  latency=1  reg_retiming=off  dbl_ovrd=off  block_type=delay
  Delay x_d2 : xbsIndex_r4/Delay  rst=off  infoeditControl=Selection of Reset will increase slice count due to use of real FFs and instead of SRLs  en=off  latency=1  reg_retiming=off  dbl_ovrd=off  block_type=delay
  Delay y1 : xbsIndex_r4/Delay  rst=off  infoeditControl=Selection of Reset will increase slice count due to use of real FFs and instead of SRLs  en=off  latency=1  reg_retiming=off  dbl_ovrd=off  block_type=delay
  Delay y2 : xbsIndex_r4/Delay  rst=off  infoeditControl=Selection of Reset will increase slice count due to use of real FFs and instead of SRLs  en=off  latency=1  reg_retiming=off  dbl_ovrd=off  block_type=delay
  Mult_a1 : xbsIndex_r4/Mult  precision=User Defined  arith_type="Signed  (2's comp)"  n_bits=16  bin_pt=15  quantization=Truncate  overflow=Wrap  en=off  latency=0  use_behavioral_HDL=off  opt=Speed  use_embedded=on  optimum_pipeline=off  pipeline=on  dbl_ovrd=off  use_rpm=on  placement_style=Triangular  block_type=mult
  Mult_a2 : xbsIndex_r4/Mult  precision=User Defined  arith_type="Signed  (2's comp)"  n_bits=16  bin_pt=15  quantization=Truncate  overflow=Wrap  en=off  latency=0  use_behavioral_HDL=off  opt=Speed  use_embedded=on  optimum_pipeline=off  pipeline=on  dbl_ovrd=off  use_rpm=on  placement_style=Triangular  block_type=mult
  Mult_b0 : xbsIndex_r4/Mult  precision=User Defined  arith_type="Signed  (2's comp)"  n_bits=16  bin_pt=15  quantization=Truncate  overflow=Wrap  en=off  latency=0  use_behavioral_HDL=off  opt=Speed  use_embedded=on  optimum_pipeline=off  pipeline=on  dbl_ovrd=off  use_rpm=on  placement_style=Triangular  block_type=mult
  Mult_b1 : xbsIndex_r4/Mult  precision=User Defined  arith_type="Signed  (2's comp)"  n_bits=16  bin_pt=15  quantization=Truncate  overflow=Wrap  en=off  latency=0  use_behavioral_HDL=off  opt=Speed  use_embedded=on  optimum_pipeline=off  pipeline=on  dbl_ovrd=off  use_rpm=on  placement_style=Triangular  block_type=mult
  Mult_b2 : xbsIndex_r4/Mult  precision=User Defined  arith_type="Signed  (2's comp)"  n_bits=16  bin_pt=15  quantization=Truncate  overflow=Wrap  en=off  latency=0  use_behavioral_HDL=off  opt=Speed  use_embedded=on  optimum_pipeline=off  pipeline=on  dbl_ovrd=off  use_rpm=on  placement_style=Triangular  block_type=mult
  Output : Outport
  wires:
  Input/1 -> Mult_b0/2, Delay x_d1/1
  Constant b0/1 -> Mult_b0/1
  Delay x_d1/1 -> Mult_b1/2, Delay x_d2/1
  Constant b1/1 -> Mult_b1/1
  Constant b2/1 -> Mult_b2/1
  Constant a1/1 -> Mult_a1/1
  Constant a2/1 -> Mult_a2/1
  Delay x_d2/1 -> Mult_b2/2
  Mult_b0/1 -> AddSub/1
  Mult_b1/1 -> AddSub/2
  AddSub/1 -> AddSub1/1
  Mult_b2/1 -> AddSub1/2
  Mult_a1/1 -> AddSub2/1
  Mult_a2/1 -> AddSub2/2
  AddSub1/1 -> AddSub3/1
  AddSub2/1 -> AddSub3/2
  AddSub3/1 -> Convert/1
  Convert/1 -> Delay y1/1
  Delay y1/1 -> Mult_a1/2, Delay y2/1
  Delay y2/1 -> Output/1, Mult_a2/2

== system vocoder_model/Channel_1/Low Pass Filter ==
  Input1 : Inport
  Add : xbsIndex_r4/AddSub  mode=Addition  use_carryin=off  use_carryout=off  en=off  latency=0  precision=User Defined  arith_type="Signed  (2's comp)"  n_bits=16  bin_pt=15  quantization=Truncate  overflow=Wrap  use_behavioral_HDL=off  hw_selection=Fabric  pipelined=off  dbl_ovrd=off  block_type=addsub
  Assert : xbsIndex_r4/Assert  assert_type=on  type_source=Explicitly  gui_display_data_type=Fixed-point  arith_type="Signed  (2's comp)"  n_bits=16  bin_pt=15  preci_type=Single  exp_width=8  frac_width=24  assert_rate=on  rate_source=Explicitly  period=1/8000  output_port=on  block_type=assert
  Delay : xbsIndex_r4/Delay  rst=off  infoeditControl=Selection of Reset will increase slice count due to use of real FFs and instead of SRLs  en=off  latency=1  reg_retiming=off  dbl_ovrd=off  block_type=delay
  Shift : xbsIndex_r4/Shift  shift_dir=Right  shift_bits=9  en=off  latency=0  precision=Full  arith_type="Signed  (2's comp)"  n_bits=16  bin_pt=14  quantization=Truncate  overflow=Wrap  dbl_ovrd=off  block_type=shift
  Subtract : xbsIndex_r4/AddSub  mode=Subtraction  use_carryin=off  use_carryout=off  en=off  latency=0  precision=User Defined  arith_type="Signed  (2's comp)"  n_bits=16  bin_pt=15  quantization=Truncate  overflow=Wrap  use_behavioral_HDL=off  hw_selection=Fabric  pipelined=off  dbl_ovrd=off  block_type=addsub
  Output1 : Outport
  wires:
  Subtract/1 -> Shift/1
  Shift/1 -> Add/1
  Add/1 -> Delay/1
  Delay/1 -> Assert/1, Output1/1
  Input1/1 -> Subtract/1
  Assert/1 -> Subtract/2, Add/2
